simulink model "Temperature_Control_System"  (R2024b)
settings: Solver=FixedStepAuto  StartTime=0.0  StopTime=10.0  FixedStep=1e-3  RelTol=1e-3
values from neighbouring files (symbols this model uses):
  K_u = K_u + 1    (= 6)    [Temp.m]
  Taw = Taw * i * 2    [Temp.m]
settings Model: Creator=LEGION  LastModifiedBy=LEGION
settings OptimizationCC: DefaultParameterBehavior=Inlined  UseDivisionForNetSlopeComputation=on  GainParamInheritBuiltInType=on  UseFloatMulNetSlope=on  InlineInvariantSignals=on  PassReuseOutputArgsAs=Individual arguments  ZeroExternalMemoryAtStartup=off  ZeroInternalMemoryAtStartup=off  NoFixptDivByZeroProtection=on  EfficientFloat2IntCast=on  LifeSpan=1  OptimizeBlockOrder=speed  DifferentSizesBufferReuse=on  EfficientTunableParamExpr=on
settings DebuggingCC: ParameterTunabilityLossMsg=error
settings HardwareCC: ProdBitPerInt=16  ProdBitPerPointer=16  ProdBitPerSizeT=16  ProdBitPerPtrDiffT=16  ProdLargestAtomicFloat=None  ProdWordSize=8  ProdLongLongMode=on  ProdHWDeviceType=Atmel->AVR
settings SFSimCC: MATLABDynamicMemAlloc=off
settings RTWCC: Description=Embedded Coder  SystemTargetFile=ert.tlc  TemplateMakefile=ert_default_tmf
settings CodeAppCC: ForceParamTrailComments=on  IgnoreCustomStorageClasses=off  OperatorAnnotations=on  SimulinkDataObjDesc=on  SFDataObjDesc=on  CustomSymbolStrGlobalVar=rt$N$M  CustomSymbolStrType=$N$M  CustomSymbolStrFcn=$N$M$F  CustomSymbolStrMacro=$N$M  InsertBlockDesc=on
settings ERTTargetCC: TargetLangStandard=C99 (ISO)  GenerateSampleERTMain=on  IncludeMdlTerminateFcn=off  CombineSignalStateStructs=on  SupportComplex=off  SupportContinuousTime=on  ERTCustomFileTemplate=example_file_process.tlc  ERTFilePackagingFormat=CompactWithDataFile

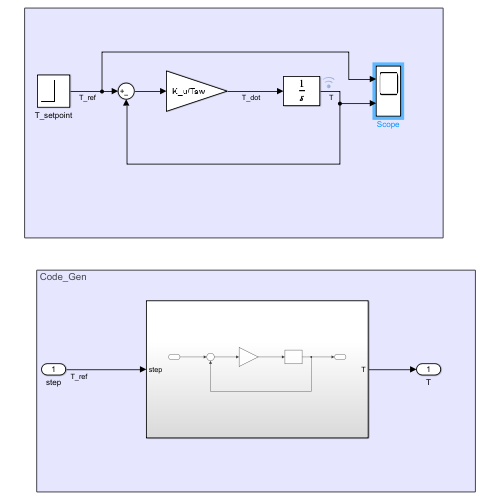
[thumbnail: Simulink's stored preview of the top-level diagram]
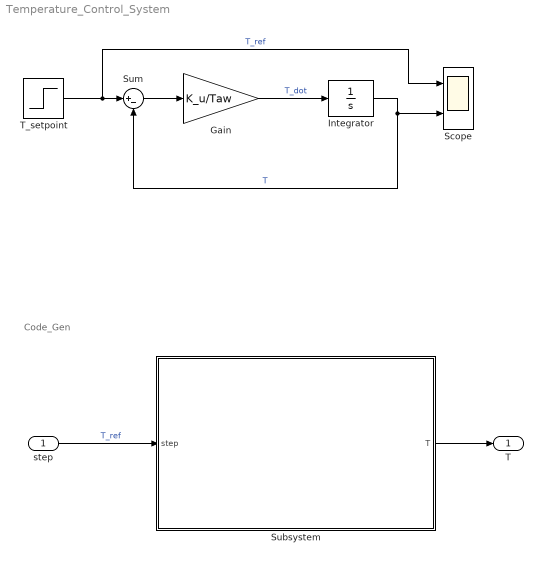
== system Temperature_Control_System ==
  note: Code_Gen
  step : Inport
  Gain : Gain  Gain=K_u/Taw
  Integrator : Integrator
  Scope : Scope  NumInputPorts=2
  Subsystem : Subsystem
  Sum : Sum  Inputs=|+-
  T_setpoint : Step  After=8  SampleTime=0
  T : Outport
  wires:
  Integrator/1 -> Sum/2, Scope/2  "T"
  T_setpoint/1 -> Scope/1, Sum/1  "T_ref"
  Sum/1 -> Gain/1
  Gain/1 -> Integrator/1  "T_dot"
  step/1 -> Subsystem/1(step)  "T_ref"
  Subsystem/1(T) -> T/1

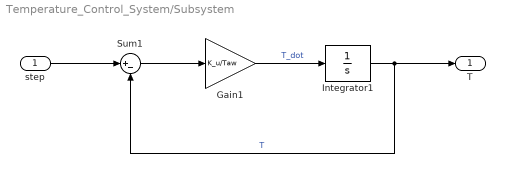
== system Temperature_Control_System/Subsystem ==
  step : Inport
  Gain1 : Gain  Gain=K_u/Taw
  Integrator1 : Integrator
  Sum1 : Sum  Inputs=|+-
  T : Outport
  wires:
  Integrator1/1 -> T/1, Sum1/2  "T"
  Gain1/1 -> Integrator1/1  "T_dot"
  Sum1/1 -> Gain1/1
  step/1 -> Sum1/1
